simulink model "sm_pmsm_model"  (R2023a)
settings: configuration reference "config" (kept outside this file)
model workspace (MATLAB code in the model file):
  | cmdLim = Simulink.Parameter;
  | cmdLim.Value = 15;
  | cmdLim.Description = 'Limit for controlling the maximum surface command angle.';
  | cmdLim.Min = 0;
  | cmdLim.Max = 90;
  | cmdLim.DocUnits = 'deg';
  | 
  | dispGain = Simulink.Parameter;
  | dispGain.Value = 0.75;
  | dispGain.Description = 'Gain applied to the displacement error.';
  | dispGain.Min = 0;
  | dispGain.Max = [];
  | dispGain.DocUnits = 'deg/sec/deg';
  | 
  | dispLim = Simulink.Parameter;
  | dispLim.Value = 30;
  | dispLim.Description = 'Limit for controlling the maximum commanded angle.';
  | dispLim.Min = 0;
  | dispLim.Max = 180;
  | dispLim.DocUnits = 'deg';
  | 
  | intGain = Simulink.Parameter;
  | intGain.Value = 0.5;
  | intGain.Description = 'Gain applied to the integral error.';
  | intGain.Min = 0;
  | intGain.Max = [];
  | intGain.DocUnits = 'deg/sec/deg/sec';
  | 
  | intLim = Simulink.Parameter;
  | intLim.Value = 5;
  | intLim.Description = 'Limit for controlling the maximum commanded angle.';
  | intLim.Min = 0;
  | intLim.Max = 90;
  | intLim.DocUnits = 'deg';
  | 
  | rateGain = Simulink.Parameter;
  | rateGain.Value = 2;
  | rateGain.Description = 'Gain applied to the rate error.';
  | rateGain.Min = 0;
  | rateGain.Max = [];
  | rateGain.DocUnits = 'deg/deg/sec';
  | 
  | rateLim = Simulink.Parameter;
  | rateLim.Value = 6;
  | rateLim.Description = 'Limit for controlling the maximum commanded angle.';
  | rateLim.Min = 0;
  | rateLim.Max = 180;
  | rateLim.DocUnits = 'deg/sec';
  | 
  | hdgGain = Simulink.Parameter;
  | hdgGain.Value = 0.015;
libraries: eeTransforms x2
settings Model: RequirementInfo={} %GIDa_fe9045fd_0412_4b6e_8206_617cc20e6fde  DataDictionary=model_config.sldd  Creator=Administrator  LastModifiedBy=Administrator
settings ConfigSetRef: SourceName=config

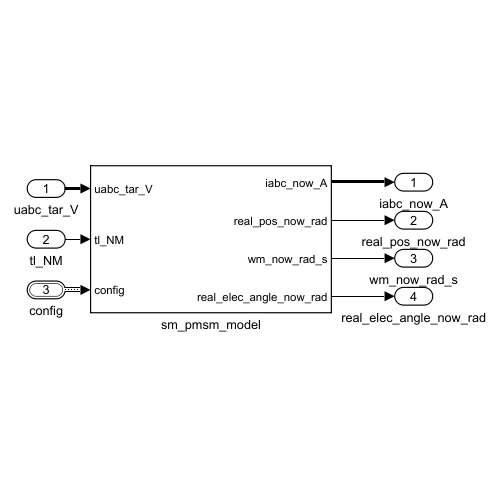
[thumbnail: Simulink's stored preview of the top-level diagram]
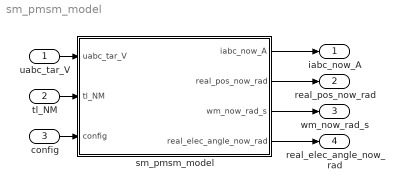
== system sm_pmsm_model ==
  uabc_tar_V : Inport
  tl_NM : Inport  Port=2
  config : Inport  Port=3  OutDataTypeStr=Bus: SimPlantConfig  BusOutputAsStruct=on
  sm_pmsm_model : Subsystem
  iabc_now_A : Outport
  real_pos_now_rad : Outport  Port=2
  wm_now_rad_s : Outport  Port=3
  real_elec_angle_now_rad : Outport  Port=4
  wires:
  sm_pmsm_model/4(real_elec_angle_now_rad) -> real_elec_angle_now_rad/1
  sm_pmsm_model/1(iabc_now_A) -> iabc_now_A/1
  uabc_tar_V/1 -> sm_pmsm_model/1(uabc_tar_V)
  tl_NM/1 -> sm_pmsm_model/2(tl_NM)
  config/1 -> sm_pmsm_model/3(config)
  sm_pmsm_model/3(wm_now_rad_s) -> wm_now_rad_s/1
  sm_pmsm_model/2(real_pos_now_rad) -> real_pos_now_rad/1

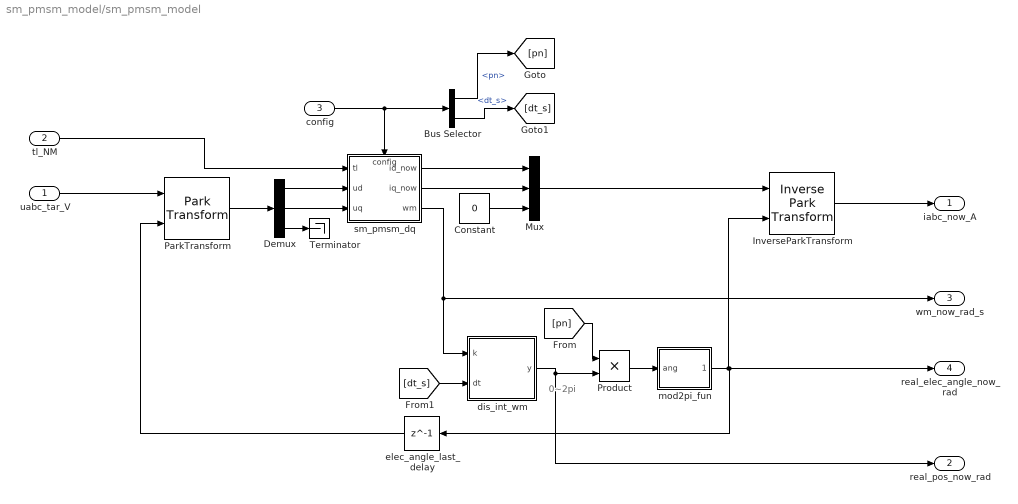
== system sm_pmsm_model/sm_pmsm_model ==
  note: 0~2pi
  uabc_tar_V : Inport  OutDataTypeStr=single  PortDimensions=3
  tl_NM : Inport  Port=2  OutDataTypeStr=single
  config : Inport  Port=3
  Bus Selector : BusSelector  OutputSignals=pn,dt_s
  Constant : Constant  Value=0  OutDataTypeStr=single  SampleTime=-1
  Demux : Demux  Outputs=3
  InverseParkTransform : eeTransforms/Inverse Park Transform  AxisAlignment=D-axis  PowerInvariant=off
      settings: LibrarySourceBlock=|
      | ee_sl_lib/Mathematical
      | Transforms/Inverse
      | Park Transform
  Mux : Mux  Inputs=3
  ParkTransform : eeTransforms/Park Transform  AxisAlignment=D-axis  PowerInvariant=off
      settings: LibrarySourceBlock=|
      | ee_sl_lib/Mathematical
      | Transforms/Park Transform
  Product : Product
  Terminator : Terminator
  dis_int_wm : Subsystem
  elec_angle_last_delay : Delay  DelayLength=1  StateName=elec_angle_last
  mod2pi_fun : MATLAB Function
  sm_pmsm_dq : Subsystem
      settings: PortSchema="{\"entries\":[{\"content\":{\"sides\":[{\"content\":{\"connectorIds\":[\"In1\",\"In2\",\"In3\"]},\"type\":\"ConnectorPlacement.EquallySpacedRectSide\",\"uuid\":\"d8cc84ce-9f3b-47a0-8bee-f47dde5345ac\"},{\"content\":{\"connectorIds\":[\"Out1\",\"Out2\",\"Out3\"],\"side\":\"RIGHT\"},\"type\":\"ConnectorPlacement.EquallySpacedRectSide\",\"uuid\":\"7a05c8dd-b607-4215-ae3a-55de450e01b9\"},{\"content\":{\"connectorIds\":[\"In4\"],\"side\":\"TOP\"},\"type\":\"ConnectorPlacement.EquallySpacedRectSide\",\"uuid\":\"29e5b71a-7e7a-40d5-8a8d-08d5a436dd58\"}]},\"type\":\"ConnectorPlacement.EquallySpacedConnector\",\"uuid\":\"95edc6c6-16f9-4a9f-9bec-fe8bb0215fcd\"}],\"packageUris\":[\"http://schema.mathworks.com/mf0/Connector/R2020b\"],\"version\":\"1.0\"}"
  iabc_now_A : Outport  OutDataTypeStr=single
  real_pos_now_rad : Outport  Port=2  OutDataTypeStr=single
  wm_now_rad_s : Outport  Port=3  OutDataTypeStr=single
  real_elec_angle_now_rad : Outport  Port=4  OutDataTypeStr=single
  wires:
  sm_pmsm_dq/2(iq_now) -> Mux/2
  InverseParkTransform/1 -> iabc_now_A/1
  Demux/3 -> Terminator/1
  sm_pmsm_dq/1(id_now) -> Mux/1
  sm_pmsm_dq/3(wm) -> dis_int_wm/1(k), wm_now_rad_s/1
  Constant/1 -> Mux/3
  Demux/2 -> sm_pmsm_dq/3(uq)
  Demux/1 -> sm_pmsm_dq/2(ud)
  dis_int_wm/1(y) -> real_pos_now_rad/1, Product/2
  tl_NM/1 -> sm_pmsm_dq/1(tl)
  ParkTransform/1 -> Demux/1
  Mux/1 -> InverseParkTransform/1
  uabc_tar_V/1 -> ParkTransform/1
  Product/1 -> mod2pi_fun/1(ang)
  mod2pi_fun/1(n_ang) -> InverseParkTransform/2, elec_angle_last_delay/1, real_elec_angle_now_rad/1
  elec_angle_last_delay/1 -> ParkTransform/2
  config/1 -> Bus Selector/1, sm_pmsm_dq/4(config)
  Bus Selector/1 -> [pn]  "<pn>"
  [pn] -> Product/1
  Bus Selector/2 -> [dt_s]  "<dt_s>"
  [dt_s] -> dis_int_wm/2(dt)

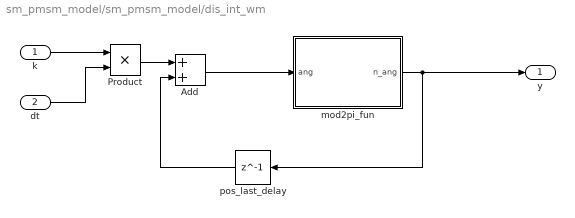
== system sm_pmsm_model/sm_pmsm_model/dis_int_wm ==
  k : Inport  OutDataTypeStr=single
  dt : Inport  Port=2
  Add : Sum
  Product : Product
  mod2pi_fun : MATLAB Function
  pos_last_delay : Delay  DelayLength=1  StateName=pos_last
  y : Outport  OutDataTypeStr=single
  wires:
  k/1 -> Product/1
  Product/1 -> Add/1
  mod2pi_fun/1(n_ang) -> y/1, pos_last_delay/1
  Add/1 -> mod2pi_fun/1(ang)
  pos_last_delay/1 -> Add/2
  dt/1 -> Product/2

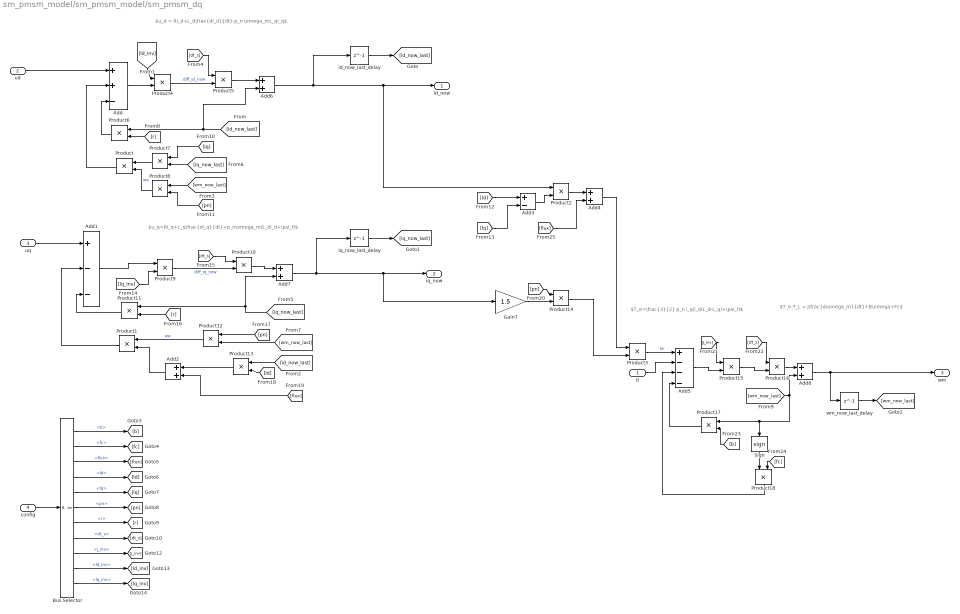
== system sm_pmsm_model/sm_pmsm_model/sm_pmsm_dq ==
  note: $u_d = Ri_d+L_d\frac{di_d}{dt}-p_n \omega_mL_qi_q$
  note: $u_q=Ri_q+L_q\frac{di_q}{dt}+p_n\omega_m(L_di_d+\psi_f)$
  note: $T_e=\frac{3}{2} p_n i_q(i_d(L_d-L_q)+\psi_f)$
  note: $T_e-T_L = J\frac{d\omega_m}{dt}+B\omega+Fc$
  tl : Inport
  ud : Inport  Port=2
  uq : Inport  Port=3
  config : Inport  Port=4
  Add : Sum  Inputs=++-
  Add1 : Sum  Inputs=+--
  Add{2,4,6..8} (5 alike) : Sum
  Add3 : Sum  Inputs=+-
  Add5 : Sum  Inputs=+---
  Bus Selector : BusSelector  OutputSignals=b,fc,flux,ld,lq,pn,r,dt_s,j_inv,ld_inv,lq_inv
  Gain7 : Gain  Gain=1.5
  Product{,1..18} (19 alike) : Product
  Sign : Signum
  id_now_last_delay : Delay  DelayLength=1  StateName=id_now_last
  iq_now_last_delay : Delay  DelayLength=1  StateName=iq_now_last
  wm_now_last_delay : Delay  DelayLength=1  StateName=wm_now_last
  id_now : Outport
  iq_now : Outport  Port=2
  wm : Outport  Port=3
  wires:
  Add6/1 -> Product2/1, id_now/1, id_now_last_delay/1
  Product7/1 -> Product/1
  Product2/1 -> Add4/1
  Sign/1 -> Product18/1
  [flux] -> Add4/2
  Product/1 -> Add/2
  Product6/1 -> Add/3
  Gain7/1 -> Product14/2
  Product13/1 -> Add2/1
  Product3/1 -> Add5/1  "te"
  Product11/1 -> Add1/3
  ud/1 -> Add/1
  [lq] -> Add3/2
  Product18/1 -> Add5/3
  Add1/1 -> Product9/1
  Product17/1 -> Add5/4
  [ld] -> Add3/1
  Product1/1 -> Add1/2
  tl/1 -> Add5/2
  Add3/1 -> Product2/2
  Add7/1 -> iq_now_last_delay/1, Gain7/1, iq_now/1
  Add2/1 -> Product1/2
  Add/1 -> Product4/2
  Add5/1 -> Product15/2
  Add8/1 -> wm/1, wm_now_last_delay/1
  id_now_last_delay/1 -> [id_now_last]
  iq_now_last_delay/1 -> [iq_now_last]
  [id_now_last] -> Product13/1
  wm_now_last_delay/1 -> [wm_now_last]
  [wm_now_last] -> Product8/1
  [wm_now_last] -> Product17/1, Sign/1, Add8/2
  [iq_now_last] -> Product7/2
  [id_now_last] -> Product6/1, Add6/2
  Product4/1 -> Product5/2  "diff_id_now"
  Product5/1 -> Add6/1
  uq/1 -> Add1/1
  Product8/1 -> Product/2  "we"
  Product12/1 -> Product1/1  "we"
  [wm_now_last] -> Product12/2
  [flux] -> Add2/2
  [iq_now_last] -> Add7/2, Product11/1
  Product10/1 -> Add7/1
  Product9/1 -> Product10/2  "diff_iq_now"
  Product16/1 -> Add8/1
  Product15/1 -> Product16/2
  Add4/1 -> Product3/1
  Product14/1 -> Product3/2
  config/1 -> Bus Selector/1
  Bus Selector/1 -> [b]  "<b>"
  Bus Selector/2 -> [fc]  "<fc>"
  Bus Selector/3 -> [flux]  "<flux>"
  Bus Selector/4 -> [ld]  "<ld>"
  Bus Selector/5 -> [lq]  "<lq>"
  Bus Selector/6 -> [pn]  "<pn>"
  Bus Selector/7 -> [r]  "<r>"
  Bus Selector/8 -> [dt_s]  "<dt_s>"
  Bus Selector/9 -> [j_inv]  "<j_inv>"
  Bus Selector/10 -> [ld_inv]  "<ld_inv>"
  Bus Selector/11 -> [lq_inv]  "<lq_inv>"
  [ld_inv] -> Product4/1
  [dt_s] -> Product5/1
  [r] -> Product6/2
  [lq] -> Product7/1
  [pn] -> Product8/2
  [lq_inv] -> Product9/2
  [dt_s] -> Product10/1
  [r] -> Product11/2
  [pn] -> Product12/1
  [ld] -> Product13/2
  [pn] -> Product14/1
  [j_inv] -> Product15/1
  [dt_s] -> Product16/1
  [b] -> Product17/2
  [fc] -> Product18/2

== matlab function sm_pmsm_model/mod2pi_fun ==
  data: ang input; n_ang output
function n_ang = mod2pi(ang)
    % 将角度限制在0到2π范围内
    TWO_PI = single(2*pi);
    n_ang = single(ang);
    while n_ang < 0
        n_ang = n_ang + TWO_PI;
    end
    while n_ang >= TWO_PI
        n_ang = n_ang - TWO_PI;
    end
end

== matlab function sm_pmsm_model/dis_int_wm/mod2pi_fun ==
  data: ang input; n_ang output
function n_ang = mod2pi(ang)
    % 将角度限制在0到2π范围内
    TWO_PI = single(2*pi);
    n_ang = single(ang);
    while n_ang < 0
        n_ang = n_ang + TWO_PI;
    end
    while n_ang >= TWO_PI
        n_ang = n_ang - TWO_PI;
    end
end
